simulink model "ValveSpec"  (R2016b)
settings: Solver=ode45  StartTime=0.0  StopTime=3600  MaxStep=5  RelTol=1e-3  EnableMultiTasking=on
undefined symbols (not defined in the file): DPConstant, DPLinear, DPQuadratic, Pressure
libraries: carnot x5, simulink x3
settings Model: Creator=drhf  LastModifiedBy=drhf
settings DataIOCC: LimitDataPoints=on  SaveFormat=Array
settings OptimizationCC: ExpressionDepthLimit=2147483647  LifeSpan=inf
settings DebuggingCC: UnderspecifiedInitializationDetection=Classic  MergeDetectMultiDrivingBlocksExec=none  SolverPrmCheckMsg=warning  StateNameClashWarn=warning  SFUnexpectedBacktrackingDiag=warning  SFNoUnconditionalDefaultTransitionDiag=warning  SFExecutionAtInitializationDiag=none
settings HardwareCC: ProdBitPerPointer=32  ProdBitPerSizeT=32  ProdBitPerPtrDiffT=32  ProdLargestAtomicFloat=None  ProdIntDivRoundTo=Undefined  ProdEndianess=Unspecified  ProdWordSize=32  ProdHWDeviceType=32-bit Generic
settings ModelReferenceCC: PropagateSignalLabelsOutOfModel=off
settings GRTTargetCC: TargetLangStandard=C89/C90 (ANSI)  GeneratePreprocessorConditionals=Disable all  CombineOutputUpdateFcns=off  GRTInterface=on
settings ConfigComp: CovMetricSettings=dw  CovHtmlReporting=on  CovSaveCumulativeToWorkspaceVar=on  CovSaveSingleToWorkspaceVar=on  CovExternalEMLEnable=off

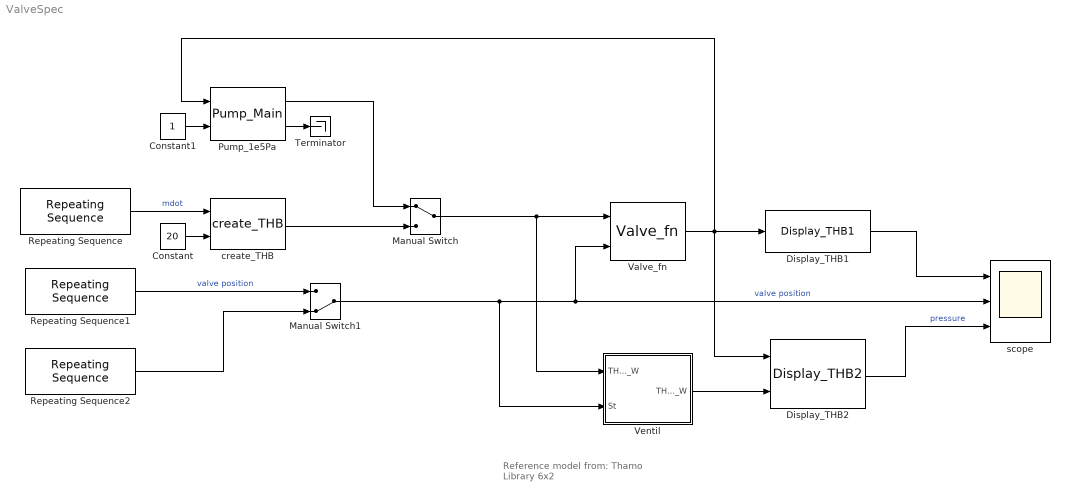
== system ValveSpec ==
  note: Reference model from:
      | Thamo Library 6x2
  Constant : Constant  Value=20
  Constant1 : Constant
  Display_THB1 : carnot/Outputs/Display_THB1  t=off  m=on  p=off  id=off  mix=off  d=off
  Display_THB2 : carnot/Outputs/Display_THB2  t=off  m=off  p=on  id=off  mix=off  d=off
  Manual Switch : ManualSwitch
  Manual Switch1 : ManualSwitch  CurrentSetting=0
  Pump_1e5Pa : carnot/Hydraulics/Pump_Main  a0=1e5  a1=0  a2=0  dia=0.025  t1=1  p0=3e5  IDchk=off  fluid_id=Water  mix=0  mix2=0  mix3=0  ua=1  mcp=500  tamb=20
  Repeating Sequence : simulink/Sources/Repeating Sequence  rep_seq_t=[0 10 20]*90  rep_seq_y=[0 0.2 0]
  Repeating Sequence1 : simulink/Sources/Repeating Sequence  rep_seq_t=[0 10 10.1 20]*90  rep_seq_y=[1 1 0.5 0.5]
  Repeating Sequence2 : simulink/Sources/Repeating Sequence  rep_seq_t=[0 1 9 11 19 20]*90  rep_seq_y=[1 1 0 0 1 1]
  Terminator : Terminator
  Valve_fn : carnot/Hydraulics/Valve_fn  ART=equal percentage  kvs=0.2*3600/1000  psi_0=0.04  dt_V=0.01
  Ventil : Subsystem  mask(Ventil){ART=gleichprozentig, kvs=0.2*3600/1000, n_0=0.04, dt_V=0.01}
      mask prompts: ART "Ventilcharakteristik"; kvs "kvs-Wert in m³/h"; n_0 "Rel. Durchflusskoeffizient"; dt_V "Ventillaufzeit in s"
      mask Help: web(fullfile(path_carnot('help'),'Valve.html'),'-helpbrowser')
      mask TypeOptions ART: linear | gleichprozentig
      mask Callback ART:
      | ART=1;
      | ART=2;
      mask Display: plot(0,10,120,180,[30,70,70,30,30]*0.8,[60,40,60,40,60]*0.8,[60,40]*0.8,[80,80]*0.8,[50,50]*0.8,[50,80]*0.8)
  create_THB : carnot/Source/Simple/create_THB  p=2e5  fluid=Water  mix=0  mix2=0  mix3=0  dia=0  hgt=0  mID=No Pressure Drop
  scope : Scope  NumInputPorts=3
  wires:
  Manual Switch1/1 -> Valve_fn/2, scope/2, Ventil/2(St)  "valve position"
  Manual Switch/1 -> Ventil/1(THB__1_W), Valve_fn/1
  Display_THB2/1 -> scope/3  "pressure"
  Constant/1 -> create_THB/2
  Repeating Sequence/1 -> create_THB/1  "mdot"
  Ventil/1(THB__2_W) -> Display_THB2/2
  Display_THB1/1 -> scope/1
  create_THB/1 -> Manual Switch/2
  Pump_1e5Pa/1 -> Manual Switch/1
  Valve_fn/1 -> Display_THB1/1, Display_THB2/1, Pump_1e5Pa/1
  Constant1/1 -> Pump_1e5Pa/2
  Pump_1e5Pa/2 -> Terminator/1
  Repeating Sequence1/1 -> Manual Switch1/1  "valve position"
  Repeating Sequence2/1 -> Manual Switch1/2

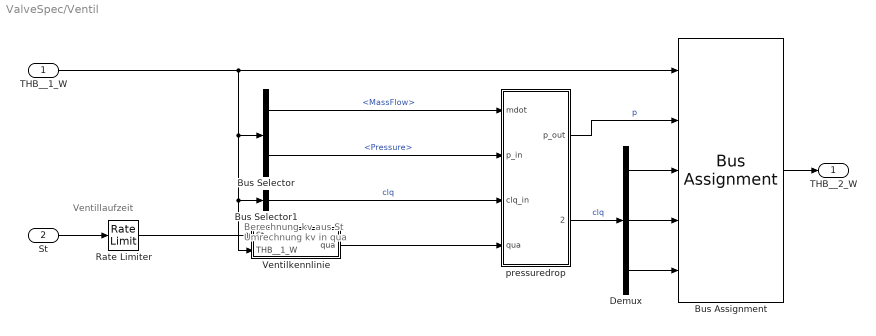
== system ValveSpec/Ventil ==
  note: Ventillaufzeit
  note: Berechnung kv aus St
      | Umrechnung kv in qua
  THB__1_W : Inport
  St : Inport  Port=2
  Bus Assignment : BusAssignment  AssignedSignals=Pressure,DPConstant,DPLinear,DPQuadratic
  Bus Selector : BusSelector  OutputSignals=MassFlow,Pressure
  Bus Selector1 : BusSelector  OutputSignals=DPConstant,DPLinear,DPQuadratic  OutputAsBus=on
  Demux : Demux  Outputs=3
  Rate Limiter : RateLimiter  RisingSlewLimit=1/dt_V  FallingSlewLimit=-1/dt_V  SampleTimeMode=inherited
  Ventilkennlinie : Subsystem
  pressuredrop : Subsystem  mask(pressure drop){}
      mask help:
      | Pressure drop according to input values of con, lin and qua:
      | dp = con + lin*mdot + qua*mdot²
      | The coefficients are also added to the correponding THB elements.
      mask Help: web(fullfile(path_carnot('help'),'Pressuredrop.html'),'-helpbrowser')
  THB__2_W : Outport
  wires:
  Demux/3 -> Bus Assignment/5
  Demux/2 -> Bus Assignment/4
  Bus Selector1/1 -> pressuredrop/3(clq_in)  "clq"
  pressuredrop/1(p_out) -> Bus Assignment/2  "p"
  Bus Selector/1 -> pressuredrop/1(mdot)  "<MassFlow>"
  Bus Selector/2 -> pressuredrop/2(p_in)  "<Pressure>"
  pressuredrop/2(clq_out) -> Demux/1  "clq"
  St/1 -> Rate Limiter/1
  THB__1_W/1 -> Bus Selector1/1, Ventilkennlinie/2(THB__1_W), Bus Selector/1, Bus Assignment/1
  Bus Assignment/1 -> THB__2_W/1
  Demux/1 -> Bus Assignment/3
  Ventilkennlinie/1(qua) -> pressuredrop/4(qua)
  Rate Limiter/1 -> Ventilkennlinie/1(St)

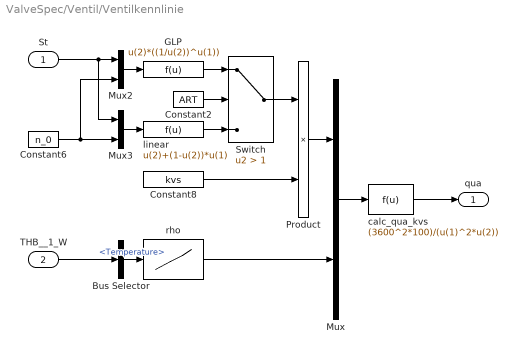
== system ValveSpec/Ventil/Ventilkennlinie ==
  St : Inport
  THB__1_W : Inport  Port=2
  Bus Selector : BusSelector  OutputSignals=Temperature
  Constant2 : Constant  Value=ART
  Constant6 : Constant  Value=n_0
  Constant8 : Constant  Value=kvs
  GLP : Fcn  Expr=u(2)*((1/u(2))^u(1))
  Mux : Mux  Inputs=2
  Mux2 : Mux  Inputs=2
  Mux3 : Mux  Inputs=2
  Product : Product
  Switch : Switch  Criteria=u2 > Threshold  Threshold=1
  calc_qua_kvs : Fcn  Expr=(3600^2*100)/(u(1)^2*u(2))
  linear : Fcn  Expr=u(2)+(1-u(2))*u(1)
  rho : Lookup_n-D  NumberOfTableDimensions=1  BreakpointsForDimension1=[0,10,20,30,40,50,60,70,80,90,100]  Table=[999.84,999.7,998.2,995.64,992.21,988.03,983.19,977.76,971.79,965.3,958.35]  InternalRulePriority=Speed  RndMeth=Simplest  InputSameDT=on
  qua : Outport
  wires:
  Bus Selector/1 -> rho/1  "<Temperature>"
  St/1 -> Mux2/1, Mux3/1
  linear/1 -> Switch/3
  Mux2/1 -> GLP/1
  Mux3/1 -> linear/1
  Constant6/1 -> Mux2/2, Mux3/2
  Constant8/1 -> Product/2
  Switch/1 -> Product/1
  Constant2/1 -> Switch/2
  GLP/1 -> Switch/1
  THB__1_W/1 -> Bus Selector/1
  calc_qua_kvs/1 -> qua/1
  Mux/1 -> calc_qua_kvs/1
  Product/1 -> Mux/1
  rho/1 -> Mux/2

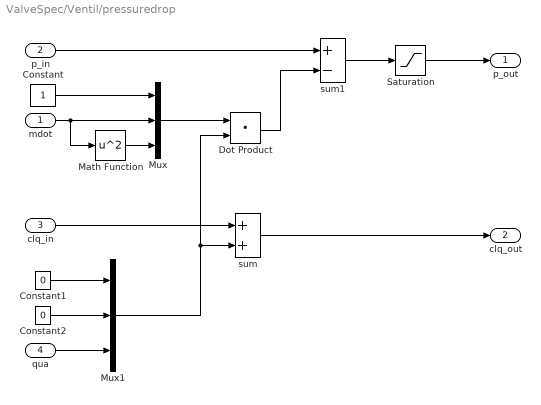
== system ValveSpec/Ventil/pressuredrop ==
  mdot : Inport
  p_in : Inport  Port=2
  clq_in : Inport  Port=3
  qua : Inport  Port=4
  Constant : Constant
  Constant1 : Constant  Value=0
  Constant2 : Constant  Value=0
  Dot Product : DotProduct  InputSameDT=on  OutDataTypeStr=Inherit: Inherit via internal rule
  Math Function : Math  Operator=square  SaturateOnIntegerOverflow=on
  Mux : Mux  Inputs=3
  Mux1 : Mux  Inputs=3
  Saturation : Saturate  UpperLimit=inf  LowerLimit=0
  sum : Sum  SaturateOnIntegerOverflow=on  InputSameDT=on  OutDataTypeStr=Inherit: Same as first input
  sum1 : Sum  Inputs=+-  SaturateOnIntegerOverflow=on  InputSameDT=on  OutDataTypeStr=Inherit: Same as first input
  p_out : Outport
  clq_out : Outport  Port=2
  wires:
  Saturation/1 -> p_out/1
  Constant/1 -> Mux/1
  mdot/1 -> Mux/2, Math Function/1
  Math Function/1 -> Mux/3
  Mux/1 -> Dot Product/1
  qua/1 -> Mux1/3
  clq_in/1 -> sum/1
  sum/1 -> clq_out/1
  Mux1/1 -> sum/2, Dot Product/2
  Dot Product/1 -> sum1/2
  p_in/1 -> sum1/1
  sum1/1 -> Saturation/1
  Constant1/1 -> Mux1/1
  Constant2/1 -> Mux1/2
